simulink model "disSG_LAS_LoadC_binary"  (R2020a)
settings: Solver=FixedStepAuto  StartTime=0.0  StopTime=inf  FixedStep=0.01  RelTol=1e-3  EnableMultiTasking=on
undefined symbols (not defined in the file or in its folder): IO392, IO397, standard
libraries: xpcutilitieslib x6, xpcseriallib x5, slrtlib x5, speedgoatlib_fpga_quadrature x4, speedgoatlib_fpga x3, hdlsllib x3, speedgoatlib_fpga_analog_io x1, speedgoatlib_IO581 x1
settings Model: SimulationMode=external  Creator=MAE-VermillionLab  LastModifiedBy=ViconLab
settings SolverCC: ConcurrentTasks=on  AutoInsertRateTranBlk=on
settings DataIOCC: SaveFormat=StructureWithTime
settings OptimizationCC: BlockReduction=off  OptimizeBlockIOStorage=off
settings HardwareCC: ProdBitPerPointer=32  ProdBitPerSizeT=32  ProdBitPerPtrDiffT=32  ProdLargestAtomicFloat=None  ProdWordSize=32  ProdLongLongMode=on  ProdHWDeviceType=Generic->32-bit x86 compatible
settings RTWCC: Description=Simulink Real-Time  SystemTargetFile=slrt.tlc  TemplateMakefile=slrt_default_tmf  CodeExecutionProfiling=on  RTWCompilerOptimization=on
settings SimulinkRealTimeCC: SupportVariableSizeSignals=on  RL32LogTETModifier=off  xPCConcurrentTasks=on

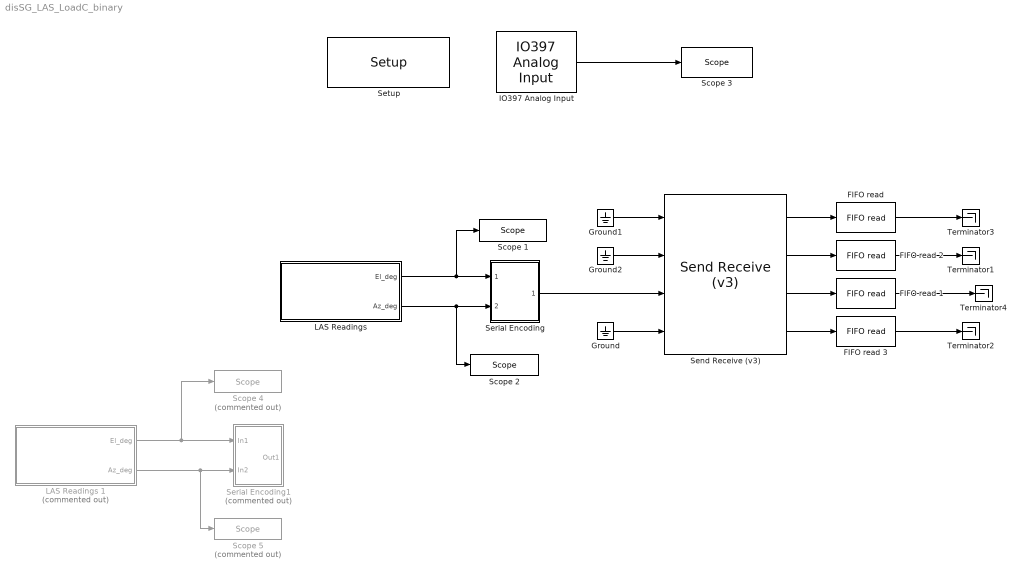
== system disSG_LAS_LoadC_binary ==
  "FIFO read " : xpcseriallib/FIFO read   maxsize=1024  minsize=1  usedelimiter=off  delimiter=13  outputtype=8 bit uint null terminated  enable=off  enableout=off  sampletime=.01
      settings: SourceProductBaseCode=XP
  FIFO read 1 : xpcseriallib/FIFO read   maxsize=1024  minsize=1  usedelimiter=off  delimiter=13  outputtype=8 bit uint null terminated  enable=off  enableout=off  sampletime=-1
      settings: SourceProductBaseCode=XP
  FIFO read 2 : xpcseriallib/FIFO read   maxsize=1024  minsize=1  usedelimiter=off  delimiter=13  outputtype=8 bit uint null terminated  enable=off  enableout=off  sampletime=.01
      settings: SourceProductBaseCode=XP
  FIFO read 3 : xpcseriallib/FIFO read   maxsize=1024  minsize=1  usedelimiter=off  delimiter=13  outputtype=8 bit uint null terminated  enable=off  enableout=off  sampletime=.01
      settings: SourceProductBaseCode=XP
  Ground : Ground
  Ground1 : Ground
  Ground2 : Ground
  IO397 Analog Input : speedgoatlib_fpga_analog_io/IO397 Analog Input  id=2  chan=1  range=+10 V  trigger=Initiator  ts=-1  pciSlot=-1  board=IO397-50k
      settings: SourceProductName=Simulink Real-Time: Speedgoat I/O Driver Library
  "LAS Readings " : Subsystem
  LAS Readings 1 : Subsystem  Commented=on
  Scope 1 : slrtlib/Displays and Logging/Scope   scopeno=1  scopetype=Target  autostart=on  viewmode=Graphical sliding  formatstr='%15.6f'  grid=on  ylimits=[0,8000]  nosamples=500  noprepostsamples=0  interleave=1  triggermode=FreeRun  triggersignal=1  trigsignalfromport=off  triggerlevel=0.0  triggerslope=Either  triggerscope=1  triggersample=0  filename=data.dat  mode=Lazy  writesize=512  autorestart=off  dynamicfilemode=off  maxwritefilesize=512*1024^2
  Scope 2 : slrtlib/Displays and Logging/Scope   scopeno=2  scopetype=Target  autostart=on  viewmode=Graphical sliding  formatstr='%15.6f'  grid=on  ylimits=[0,8000]  nosamples=500  noprepostsamples=0  interleave=1  triggermode=FreeRun  triggersignal=1  trigsignalfromport=off  triggerlevel=0.0  triggerslope=Either  triggerscope=1  triggersample=0  filename=data.dat  mode=Lazy  writesize=512  autorestart=off  dynamicfilemode=off  maxwritefilesize=512*1024^2
  Scope 3 : slrtlib/Displays and Logging/Scope   scopeno=3  scopetype=Target  autostart=on  viewmode=Numerical  formatstr='%15.6f'  grid=on  ylimits=[0,0]  nosamples=2000  noprepostsamples=0  interleave=1  triggermode=FreeRun  triggersignal=1  trigsignalfromport=off  triggerlevel=0.0  triggerslope=Either  triggerscope=1  triggersample=0  filename=data.dat  mode=Lazy  writesize=512  autorestart=off  dynamicfilemode=off  maxwritefilesize=512*1024^2
  Scope 4 : slrtlib/Displays and Logging/Scope   Commented=on  scopeno=1  scopetype=Target  autostart=on  viewmode=Numerical  formatstr='%15.6f'  grid=on  ylimits=[0,0]  nosamples=2000  noprepostsamples=0  interleave=1  triggermode=FreeRun  triggersignal=1  trigsignalfromport=off  triggerlevel=0.0  triggerslope=Either  triggerscope=1  triggersample=0  filename=data.dat  mode=Lazy  writesize=512  autorestart=off  dynamicfilemode=off  maxwritefilesize=512*1024^2
  Scope 5 : slrtlib/Displays and Logging/Scope   Commented=on  scopeno=2  scopetype=Target  autostart=on  viewmode=Numerical  formatstr='%15.6f'  grid=on  ylimits=[0,0]  nosamples=2000  noprepostsamples=0  interleave=1  triggermode=FreeRun  triggersignal=1  trigsignalfromport=off  triggerlevel=0.0  triggerslope=Either  triggerscope=1  triggersample=0  filename=data.dat  mode=Lazy  writesize=512  autorestart=off  dynamicfilemode=off  maxwritefilesize=512*1024^2
  "Send Receive (v3) " : speedgoatlib_IO581/Send Receive (v3)   parModuleId=1  parSlot=-1  parModuleType=IO581  parTransceiver12=RS485 Half-Duplex  parTransceiver34=RS485 Half-Duplex  parTransceiver1=RS485 Half-Duplex  parAutoTurnaround1=off  parTurnaroundDelay1=0  parStandardBaud1=on  parBaudrate1=38400  parBaudDivisor1=1  parSamplingRate1=16x (standard)  parPrescale1=off  parCalcBaud1=7812500  parParity1=None  parDataBits1=8  parStopBits1=1  parTxTrigLvl1=1  parRxTrigLvl1=1  parHandshake1=none  parRtsHysteresis1=0  parXon1=17  parXoff1=19  parTxSwFifoSize1=1024  parTxSwFifoType1=8 bit uint null terminated  parRxSwFifoSize1=1024  parTransceiver2=RS485 Half-Duplex  parAutoTurnaround2=off  parTurnaroundDelay2=0  parStandardBaud2=on  parBaudrate2=115200  parBaudDivisor2=1  parSamplingRate2=16x (standard)  parPrescale2=off  parCalcBaud2=7812500  parParity2=None  parDataBits2=8  parStopBits2=1  parTxTrigLvl2=1  parRxTrigLvl2=1  parHandshake2=none  parRtsHysteresis2=0  parXon2=17  parXoff2=19  parTxSwFifoSize2=1024  parTxSwFifoType2=8 bit uint null terminated  parRxSwFifoSize2=1024  parTransceiver3=RS485 Half-Duplex  parAutoTurnaround3=off  parTurnaroundDelay3=0  parStandardBaud3=on  parBaudrate3=115200  parBaudDivisor3=1  parSamplingRate3=16x (standard)  parPrescale3=off  parCalcBaud3=7812500  parParity3=None  parDataBits3=8  parStopBits3=1  parTxTrigLvl3=1  parRxTrigLvl3=1  parHandshake3=none  parRtsHysteresis3=0  parXon3=17  parXoff3=19  parTxSwFifoSize3=1024  parTxSwFifoType3=8 bit uint null terminated  parRxSwFifoSize3=1024  parTransceiver4=RS485 Half-Duplex  parAutoTurnaround4=off  parTurnaroundDelay4=0  parStandardBaud4=on  parBaudrate4=1382400  parBaudDivisor4=1  parSamplingRate4=16x (standard)  parPrescale4=off  parCalcBaud4=7812500  parParity4=None  parDataBits4=8  parStopBits4=1  parTxTrigLvl4=10  parRxTrigLvl4=1  parHandshake4=none  parRtsHysteresis4=0  parXon4=17  parXoff4=19  parTxSwFifoSize4=1024  parTxSwFifoType4=8 bit uint null terminated  parRxSwFifoSize4=1024
      settings: SourceProductName=Simulink Real-Time: Speedgoat Library
  Serial Encoding : Subsystem
  Serial Encoding1 : Subsystem  Commented=on
  Setup : speedgoatlib_fpga/Setup/Setup  board=IO397-50k  id=2  device_id=1  frontIO=None  rearIO=None  bitstreamFile=speedgoat_IO397_50k_CI_02113  rev=1.0  timestamp_string=21/04/20 11:41:53  fpgaFreq=75 MHz  fpgaTick=13.33 ns  ProgSpiFlash=off  ProgBPIFlash=off  pciSlot=-1  PullRPort0=pull-up 3.3V  VioPort0=3.3V  PullRPort1=pull-up 3.3V  VioPort1=3.3V  PullRPort2=pull-up 3.3V  VioPort2=3.3V  PullRPort3=pull-up 3.3V  VioPort3=3.3V  PullRPort4=pull-up 3.3V  VioPort4=3.3V  PullRPort5=pull-up 3.3V  VioPort5=3.3V  PullRPort6=pull-up 3.3V  VioPort6=3.3V  PullRPort15=pull-up 3.3V  PullRPort31=pull-up 3.3V  PullRPort47=pull-up 3.3V  PullRPort63=pull-up 3.3V
      settings: SourceProductName=Simulink Real-Time: Speedgoat Library
  Terminator{1..4} (4 alike) : Terminator
  wires:
  Ground1/1 -> "Send Receive (v3) "/1
  FIFO read 1/1 -> Terminator4/1
  Ground2/1 -> "Send Receive (v3) "/2
  "Send Receive (v3) "/4 -> FIFO read 3/1
  "Send Receive (v3) "/2 -> FIFO read 2/1
  "Send Receive (v3) "/1 -> "FIFO read "/1
  "Send Receive (v3) "/3 -> FIFO read 1/1
  "LAS Readings "/1(El_deg) -> Scope 1/1, Serial Encoding/1("Serial_El ")
  "LAS Readings "/2(Az_deg) -> Scope 2/1, Serial Encoding/2(Serial_Az)
  IO397 Analog Input/1 -> Scope 3/1
  "FIFO read "/1 -> Terminator3/1
  FIFO read 2/1 -> Terminator1/1
  FIFO read 3/1 -> Terminator2/1
  LAS Readings 1/1(El_deg) -> Scope 4/1, Serial Encoding1/1(In1)
  LAS Readings 1/2(Az_deg) -> Scope 5/1, Serial Encoding1/2(In2)
  Ground/1 -> "Send Receive (v3) "/4
  Serial Encoding/1(Out1) -> "Send Receive (v3) "/3

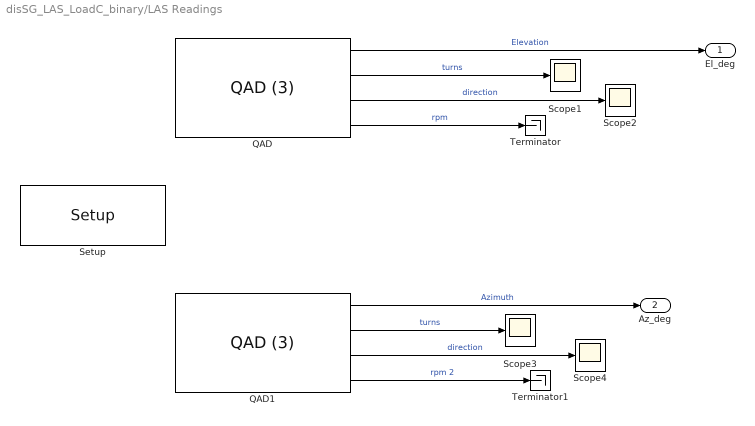
== system disSG_LAS_LoadC_binary/LAS Readings  ==
  QAD : speedgoatlib_fpga_quadrature/QAD (3)  id=1  board=IO392-50k  chan=[2]  resetOnStart=on  ts=0.01  pciSlot=-1  operatingMode=Quadrature decoder  indexControlMode=Reset on index  resolution=4x  stepsPerRevolution=[8191]  latchMode=Disabled  interpolatePosition=off  invertAB=off  showClearPositionInput=off  showClearIndexFoundInput=off  showPositionOutput=on  showTurnOutput=on  showSpeedOutput=on  showDirectionOutput=on  showIndexFoundOutput=off
      settings: SourceProductName=Simulink Real-Time: Speedgoat I/O Driver Library
  QAD1 : speedgoatlib_fpga_quadrature/QAD (3)  id=1  board=IO392-50k  chan=[1]  resetOnStart=on  ts=0.01  pciSlot=-1  operatingMode=Quadrature decoder  indexControlMode=Reset on index  resolution=4x  stepsPerRevolution=[8191]  latchMode=Disabled  interpolatePosition=off  invertAB=off  showClearPositionInput=off  showClearIndexFoundInput=off  showPositionOutput=on  showTurnOutput=on  showSpeedOutput=on  showDirectionOutput=on  showIndexFoundOutput=off
      settings: SourceProductName=Simulink Real-Time: Speedgoat I/O Driver Library
  Scope{1..4} (4 alike) : Scope
  Setup : speedgoatlib_fpga/Setup/Setup  board=IO392-50k  id=1  device_id=1  frontIO=None  rearIO=None  bitstreamFile=speedgoat_IO392_50k_CI_02244  rev=1.0  timestamp_string=07/12/20 12:10:05  fpgaFreq=75 MHz  fpgaTick=13.33 ns  ProgSpiFlash=off  ProgBPIFlash=off  pciSlot=-1  PullRPort0=pull-up 3.3V  VioPort0=3.3V  PullRPort1=pull-up 3.3V  VioPort1=3.3V  PullRPort2=pull-up 3.3V  VioPort2=3.3V  PullRPort3=pull-up 3.3V  VioPort3=3.3V  PullRPort4=pull-up 3.3V  VioPort4=3.3V  PullRPort5=pull-up 3.3V  VioPort5=3.3V  PullRPort6=pull-up 3.3V  VioPort6=3.3V  PullRPort15=pull-up 3.3V  PullRPort31=pull-up 3.3V  PullRPort47=pull-up 3.3V  PullRPort63=pull-up 3.3V
      settings: SourceProductName=Simulink Real-Time: Speedgoat Library
  Terminator : Terminator
  Terminator1 : Terminator
  El_deg : Outport
  Az_deg : Outport  Port=2
  wires:
  QAD1/2 -> Scope3/1  "turns"
  QAD/3 -> Scope2/1  "direction"
  QAD/4 -> Terminator/1  "rpm"
  QAD1/3 -> Scope4/1  "direction"
  QAD/1 -> El_deg/1  "Elevation"
  QAD/2 -> Scope1/1  "turns"
  QAD1/1 -> Az_deg/1  "Azimuth"
  QAD1/4 -> Terminator1/1  "rpm 2"

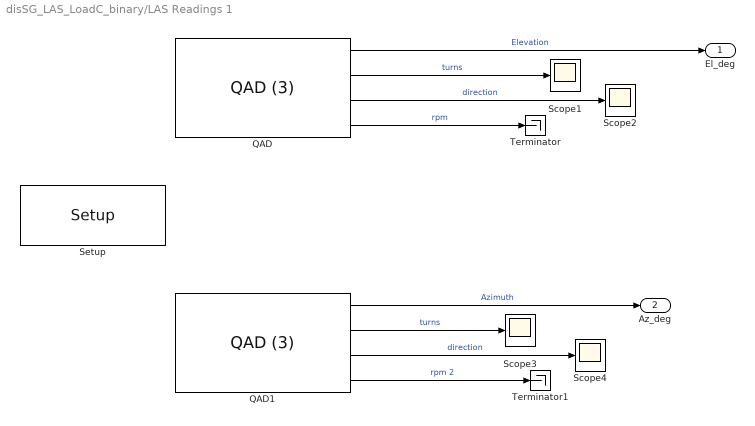
== system disSG_LAS_LoadC_binary/LAS Readings 1 ==
  QAD : speedgoatlib_fpga_quadrature/QAD (3)  id=1  board=IO392-50k  chan=[2]  resetOnStart=on  ts=0.01  pciSlot=-1  operatingMode=Quadrature decoder  indexControlMode=Reset on index  resolution=4x  stepsPerRevolution=[8191]  latchMode=Disabled  interpolatePosition=off  invertAB=off  showClearPositionInput=off  showClearIndexFoundInput=off  showPositionOutput=on  showTurnOutput=on  showSpeedOutput=on  showDirectionOutput=on  showIndexFoundOutput=off
      settings: SourceProductName=Simulink Real-Time: Speedgoat I/O Driver Library
  QAD1 : speedgoatlib_fpga_quadrature/QAD (3)  id=1  board=IO392-50k  chan=[1]  resetOnStart=on  ts=0.01  pciSlot=-1  operatingMode=Quadrature decoder  indexControlMode=Reset on index  resolution=4x  stepsPerRevolution=[8191]  latchMode=Disabled  interpolatePosition=off  invertAB=off  showClearPositionInput=off  showClearIndexFoundInput=off  showPositionOutput=on  showTurnOutput=on  showSpeedOutput=on  showDirectionOutput=on  showIndexFoundOutput=off
      settings: SourceProductName=Simulink Real-Time: Speedgoat I/O Driver Library
  Scope{1..4} (4 alike) : Scope
  Setup : speedgoatlib_fpga/Setup/Setup  board=IO392-50k  id=1  device_id=1  frontIO=None  rearIO=None  bitstreamFile=speedgoat_IO392_50k_CI_02244  rev=1.0  timestamp_string=07/12/20 12:10:05  fpgaFreq=75 MHz  fpgaTick=13.33 ns  ProgSpiFlash=off  ProgBPIFlash=off  pciSlot=-1  PullRPort0=pull-up 3.3V  VioPort0=3.3V  PullRPort1=pull-up 3.3V  VioPort1=3.3V  PullRPort2=pull-up 3.3V  VioPort2=3.3V  PullRPort3=pull-up 3.3V  VioPort3=3.3V  PullRPort4=pull-up 3.3V  VioPort4=3.3V  PullRPort5=pull-up 3.3V  VioPort5=3.3V  PullRPort6=pull-up 3.3V  VioPort6=3.3V  PullRPort15=pull-up 3.3V  PullRPort31=pull-up 3.3V  PullRPort47=pull-up 3.3V  PullRPort63=pull-up 3.3V
      settings: SourceProductName=Simulink Real-Time: Speedgoat Library
  Terminator : Terminator
  Terminator1 : Terminator
  El_deg : Outport
  Az_deg : Outport  Port=2
  wires:
  QAD1/4 -> Terminator1/1  "rpm 2"
  QAD1/1 -> Az_deg/1  "Azimuth"
  QAD/2 -> Scope1/1  "turns"
  QAD/1 -> El_deg/1  "Elevation"
  QAD1/3 -> Scope4/1  "direction"
  QAD/4 -> Terminator/1  "rpm"
  QAD/3 -> Scope2/1  "direction"
  QAD1/2 -> Scope3/1  "turns"

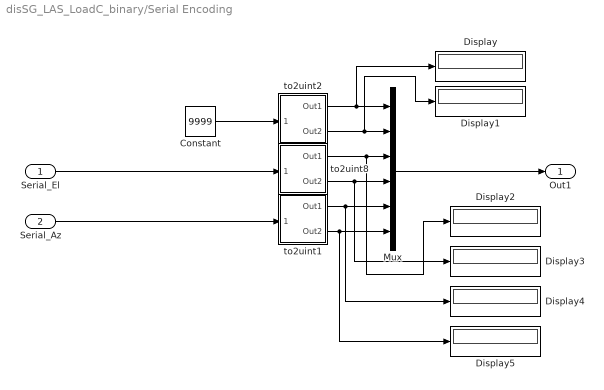
== system disSG_LAS_LoadC_binary/Serial Encoding ==
  "Serial_El " : Inport
  Serial_Az : Inport  Port=2
  Constant : Constant  Value=9999  OutDataTypeStr=uint16
  Display{,1..5} (6 alike) : Display
      settings: Format=hex (Stored Integer)
  Mux : Mux  Inputs=6
  to2uint1 : Subsystem
  to2uint2 : Subsystem
  to2uint8 : Subsystem
  Out1 : Outport
  wires:
  "Serial_El "/1 -> to2uint8/1(" ")
  Serial_Az/1 -> to2uint1/1(" ")
  Constant/1 -> to2uint2/1(" ")
  to2uint2/1(Out1) -> Display/1, Mux/1
  to2uint2/2(Out2) -> Display1/1, Mux/2
  to2uint8/1(Out1) -> Display2/1, Mux/3
  to2uint8/2(Out2) -> Display3/1, Mux/4
  to2uint1/1(Out1) -> Display4/1, Mux/5
  to2uint1/2(Out2) -> Display5/1, Mux/6
  Mux/1 -> Out1/1

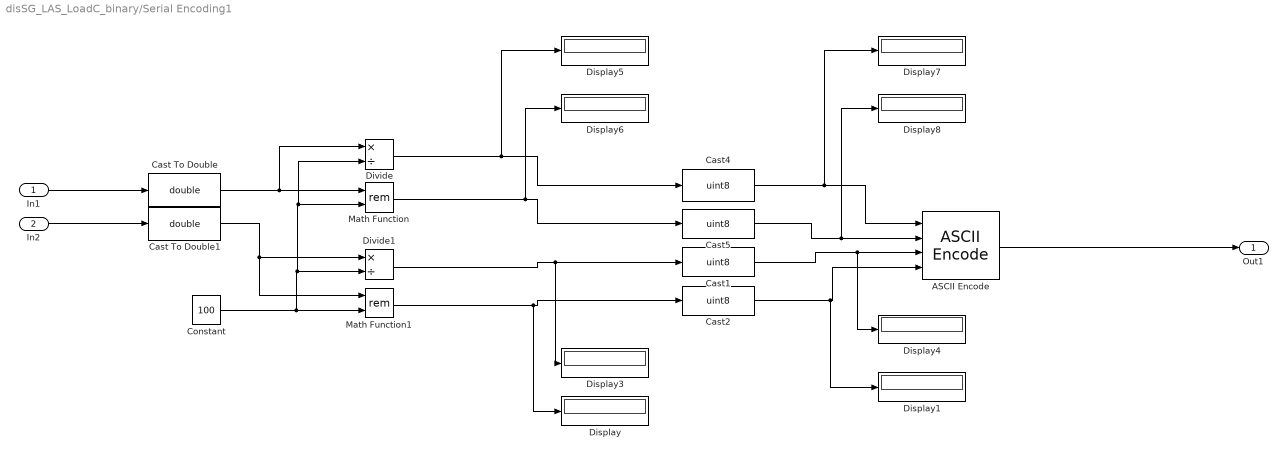
== system disSG_LAS_LoadC_binary/Serial Encoding1 ==
  In1 : Inport
  In2 : Inport  Port=2
  "ASCII Encode " : xpcseriallib/ASCII Encode   format=A%d\r\nB%d\r\nC%d\r\nD%d\r\n  nvars=4  maxlength=256  vartypes={ 'uint8' }
      settings: SourceProductBaseCode=XP
  Cast To Double : DataTypeConversion  OutDataTypeStr=double
  Cast To Double1 : DataTypeConversion  OutDataTypeStr=double
  Cast{1..2,4..5} (4 alike) : DataTypeConversion  OutDataTypeStr=uint8
  Constant : Constant  Value=100
  Display{,1,3..8} (8 alike) : Display
  Divide : Product  Inputs=*/
  Divide1 : Product  Inputs=*/
  Math Function : Math  Operator=rem  OutputSignalType=real  SaturateOnIntegerOverflow=on
  Math Function1 : Math  Operator=rem  OutputSignalType=real  SaturateOnIntegerOverflow=on
  Out1 : Outport
  wires:
  Divide/1 -> Display5/1, Cast4/1
  Math Function/1 -> Display6/1, Cast5/1
  Cast2/1 -> Display1/1, "ASCII Encode "/4
  Constant/1 -> Divide/2, Math Function/2, Divide1/2, Math Function1/2
  In1/1 -> Cast To Double/1
  Math Function1/1 -> Display/1, Cast2/1
  Cast4/1 -> Display7/1, "ASCII Encode "/1
  Cast To Double1/1 -> Math Function1/1, Divide1/1
  Divide1/1 -> Display3/1, Cast1/1
  Cast1/1 -> Display4/1, "ASCII Encode "/3
  "ASCII Encode "/1 -> Out1/1
  Cast5/1 -> Display8/1, "ASCII Encode "/2
  In2/1 -> Cast To Double1/1
  Cast To Double/1 -> Math Function/1, Divide/1

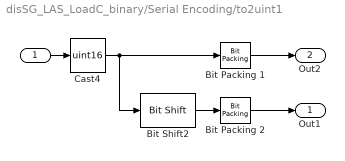
== system disSG_LAS_LoadC_binary/Serial Encoding/to2uint1 ==
  " " : Inport
  Bit Packing 1 : xpcutilitieslib/Bit Packing   MaskBitPatterns={[0:7]}  MaskPackDataType=uint8  MaskPackDataSize=[1]
      settings: SourceProductBaseCode=XP
  Bit Packing 2 : xpcutilitieslib/Bit Packing   MaskBitPatterns={[0:7]}  MaskPackDataType=uint8  MaskPackDataSize=[1]
      settings: SourceProductBaseCode=XP
  Bit Shift2 : hdlsllib/Logic and Bit Operations/Bit Shift  mode=Shift Right Arithmetic  N=8
  Cast4 : DataTypeConversion  OutDataTypeStr=uint16
  Out1 : Outport
  Out2 : Outport  Port=2
  wires:
  " "/1 -> Cast4/1
  Cast4/1 -> Bit Packing 1/1, Bit Shift2/1
  Bit Shift2/1 -> Bit Packing 2/1
  Bit Packing 2/1 -> Out1/1
  Bit Packing 1/1 -> Out2/1

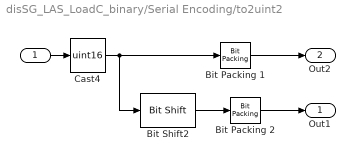
== system disSG_LAS_LoadC_binary/Serial Encoding/to2uint2 ==
  " " : Inport
  Bit Packing 1 : xpcutilitieslib/Bit Packing   MaskBitPatterns={[0:7]}  MaskPackDataType=uint8  MaskPackDataSize=[1]
      settings: SourceProductBaseCode=XP
  Bit Packing 2 : xpcutilitieslib/Bit Packing   MaskBitPatterns={[0:7]}  MaskPackDataType=uint8  MaskPackDataSize=[1]
      settings: SourceProductBaseCode=XP
  Bit Shift2 : hdlsllib/Logic and Bit Operations/Bit Shift  mode=Shift Right Arithmetic  N=8
  Cast4 : DataTypeConversion  OutDataTypeStr=uint16
  Out1 : Outport
  Out2 : Outport  Port=2
  wires:
  " "/1 -> Cast4/1
  Cast4/1 -> Bit Packing 1/1, Bit Shift2/1
  Bit Shift2/1 -> Bit Packing 2/1
  Bit Packing 2/1 -> Out1/1
  Bit Packing 1/1 -> Out2/1

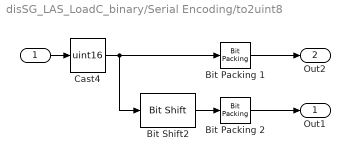
== system disSG_LAS_LoadC_binary/Serial Encoding/to2uint8 ==
  " " : Inport
  Bit Packing 1 : xpcutilitieslib/Bit Packing   MaskBitPatterns={[0:7]}  MaskPackDataType=uint8  MaskPackDataSize=[1]
      settings: SourceProductBaseCode=XP
  Bit Packing 2 : xpcutilitieslib/Bit Packing   MaskBitPatterns={[0:7]}  MaskPackDataType=uint8  MaskPackDataSize=[1]
      settings: SourceProductBaseCode=XP
  Bit Shift2 : hdlsllib/Logic and Bit Operations/Bit Shift  mode=Shift Right Arithmetic  N=8
  Cast4 : DataTypeConversion  OutDataTypeStr=uint16
  Out1 : Outport
  Out2 : Outport  Port=2
  wires:
  Bit Shift2/1 -> Bit Packing 2/1
  Cast4/1 -> Bit Shift2/1, Bit Packing 1/1
  " "/1 -> Cast4/1
  Bit Packing 2/1 -> Out1/1
  Bit Packing 1/1 -> Out2/1
